simulink model "ADIA"  (R2018b)
settings: Solver=FixedStepDiscrete  StartTime=0.0  StopTime=10.0  FixedStep=0.02  RelTol=1e-3
undefined symbols (not defined in the file or in its folder): ACC_State_Active, ACC_State_BrakeOnly, ACC_State_Suspended, ACC_State_WaitingRise, ADAS_AEBBrakingProg, ADAS_DeclControlReq, ADAS_DriveOff, ADAS_ESCHoldReq_NotHold, ADASDecType_ACC, ADASDecType_AEB, ADIA_ACC_Acceleration_OOR_DecCount_C, ADIA_ACC_Acceleration_OOR_Duration_C, ADIA_ACC_Acceleration_OOR_IncCount_C, ADIA_ACC_Acceleration_OOR_LLim_C, ADIA_ACC_Acceleration_OOR_ULim_C, ADIA_ACC_AccelTrqReq_MixedDia_ULim_C, ADIA_ACC_AccelTrqReq_ULim_C, ADIA_ACC_Deceleration_Mixed_ULim_C, ADIA_ACC_Deceleration_OOR_DecCount_C, ADIA_ACC_Deceleration_OOR_Duration_C, ADIA_ACC_Deceleration_OOR_IncCount_C, ADIA_ACC_Deceleration_OOR_LLim_C, ADIA_ACC_Deceleration_OOR_ULim_C, ADIA_ACC_DriveOff_Distance_C, ADIA_ACC_DriveOff_TimeLim_C, ADIA_ACC_ReqMixed_DecCount_C, ADIA_ACC_ReqMixed_Duration_C, ADIA_ACC_ReqMixed_IncCount_C, ADIA_AccPedalRaw_MaxLim_C, ADIA_AccPedalRaw_MinLim_C, ADIA_ADAS_HoldDecReq_Set_C, ADIA_ADAS_HoldRConfirm_TimeLim_C, ADIA_ADAS_HoldVehSpd_Lim_C, ADIA_AEB_VehSpdDec_LLim_C, ADIA_AEB_VehSpdDec_ULim_C, ADIA_ASWFault_OvrdEn_C, ADIA_ASWFault_OvrdValue_C, ADIA_BatteryOutOfRange_DecCount_C, ADIA_BatteryOutOfRange_Duration_C, ADIA_BatteryOutOfRange_IncCount_C, ADIA_BattVolt_MaxLim_C, ADIA_BattVolt_MinLim_C, ADIA_BCM3_33C_InvBrkLight_DecCount_C, ADIA_BCM3_33C_InvBrkLight_Duration_C, ADIA_BCM3_33C_InvBrkLight_IncCount_C, ADIA_BCM_BattVolt_OvrdEn_C, ADIA_BCM_BattVolt_OvrdVal_C, ADIA_BCM_BrakeLampStaus_OvrdEn_C, ADIA_BCM_BrakeLampStaus_OvrdVal_C, ADIA_BCM_CHMSLStaus_OvrdEn_C, ADIA_BCM_CHMSLStaus_OvrdVal_C, ADIA_BCM_LeftTurnSwSt_OvrdEn_C, ADIA_BCM_LeftTurnSwSt_OvrdVal_C, ADIA_BCM_RightTurnSwSt_OvrdEn_C, ADIA_BCM_RightTurnSwSt_OvrdVal_C, ADIA_BCM_TurnSwFailure_DecCount_C, ADIA_BCM_TurnSwFailure_Duration_C, ADIA_BCM_TurnSwFailure_IncCount_C, ADIA_BSWFault_Ignore_C, ADIA_BSWFault_OvrdEn_C ... (+281)
libraries: simulink x208
(part 8 of 10)

== system ADIA/ADAS_Diagnostics/Diagnostics_Processing/Subsystem3/16Bits_Set1/8Bits_Set1 ==
  Bit1 : Inport  OutDataTypeStr=boolean
  Bit2 : Inport  Port=2  OutDataTypeStr=boolean
  Bit3 : Inport  Port=3  OutDataTypeStr=boolean
  Bit4 : Inport  Port=4  OutDataTypeStr=boolean
  Bit5 : Inport  Port=5  OutDataTypeStr=boolean
  Bit6 : Inport  Port=6  OutDataTypeStr=boolean
  Bit7 : Inport  Port=7  OutDataTypeStr=boolean
  Bit8 : Inport  Port=8  OutDataTypeStr=boolean
  Bit Clear : simulink/Logic and Bit Operations/Bit Clear  iBit=0
      settings: SourceProductName=Simulink  SourceProductBaseCode=SL
  Bit Clear1 : simulink/Logic and Bit Operations/Bit Clear  iBit=1
      settings: SourceProductName=Simulink  SourceProductBaseCode=SL
  Bit Clear2 : simulink/Logic and Bit Operations/Bit Clear  iBit=2
      settings: SourceProductName=Simulink  SourceProductBaseCode=SL
  Bit Clear3 : simulink/Logic and Bit Operations/Bit Clear  iBit=3
      settings: SourceProductName=Simulink  SourceProductBaseCode=SL
  Bit Clear4 : simulink/Logic and Bit Operations/Bit Clear  iBit=5
      settings: SourceProductName=Simulink  SourceProductBaseCode=SL
  Bit Clear5 : simulink/Logic and Bit Operations/Bit Clear  iBit=4
      settings: SourceProductName=Simulink  SourceProductBaseCode=SL
  Bit Clear6 : simulink/Logic and Bit Operations/Bit Clear  iBit=6
      settings: SourceProductName=Simulink  SourceProductBaseCode=SL
  Bit Clear7 : simulink/Logic and Bit Operations/Bit Clear  iBit=7
      settings: SourceProductName=Simulink  SourceProductBaseCode=SL
  Bit Set : simulink/Logic and Bit Operations/Bit Set  iBit=0
      settings: SourceProductName=Simulink  SourceProductBaseCode=SL
  Bit Set1 : simulink/Logic and Bit Operations/Bit Set  iBit=1
      settings: SourceProductName=Simulink  SourceProductBaseCode=SL
  Bit Set2 : simulink/Logic and Bit Operations/Bit Set  iBit=2
      settings: SourceProductName=Simulink  SourceProductBaseCode=SL
  Bit Set3 : simulink/Logic and Bit Operations/Bit Set  iBit=3
      settings: SourceProductName=Simulink  SourceProductBaseCode=SL
  Bit Set4 : simulink/Logic and Bit Operations/Bit Set  iBit=4
      settings: SourceProductName=Simulink  SourceProductBaseCode=SL
  Bit Set5 : simulink/Logic and Bit Operations/Bit Set  iBit=5
      settings: SourceProductName=Simulink  SourceProductBaseCode=SL
  Bit Set6 : simulink/Logic and Bit Operations/Bit Set  iBit=6
      settings: SourceProductName=Simulink  SourceProductBaseCode=SL
  Bit Set7 : simulink/Logic and Bit Operations/Bit Set  iBit=7
      settings: SourceProductName=Simulink  SourceProductBaseCode=SL
  Delay : Delay  DelayLength=1  InitialCondition=0
  Switch{1..8} (8 alike) : Switch  Criteria=u2 > Threshold
  Index_8Bits : Outport  OutDataTypeStr=uint8
  wires:
  Bit Clear7/1 -> Switch8/3
  Bit Clear6/1 -> Switch7/3
  Bit Clear5/1 -> Switch5/3
  Bit Clear4/1 -> Switch6/3
  Bit Clear3/1 -> Switch4/3
  Bit Clear2/1 -> Switch3/3
  Bit Clear1/1 -> Switch2/3
  Bit Clear/1 -> Switch1/3
  Bit Set4/1 -> Switch5/1
  Bit Set2/1 -> Switch3/1
  Switch4/1 -> Bit Set4/1, Bit Clear5/1
  Switch6/1 -> Bit Set6/1, Bit Clear6/1
  Bit Set5/1 -> Switch6/1
  Switch7/1 -> Bit Set7/1, Bit Clear7/1
  Switch2/1 -> Bit Set2/1, Bit Clear2/1
  Bit Set3/1 -> Switch4/1
  Bit Set/1 -> Switch1/1
  Switch3/1 -> Bit Set3/1, Bit Clear3/1
  Bit7/1 -> Switch7/2
  Bit8/1 -> Switch8/2
  Bit Set6/1 -> Switch7/1
  Bit5/1 -> Switch5/2
  Bit6/1 -> Switch6/2
  Bit3/1 -> Switch3/2
  Bit Set1/1 -> Switch2/1
  Delay/1 -> Bit Set/1, Bit Clear/1
  Switch5/1 -> Bit Set5/1, Bit Clear4/1
  Bit2/1 -> Switch2/2
  Switch1/1 -> Bit Set1/1, Bit Clear1/1
  Switch8/1 -> Delay/1, Index_8Bits/1
  Bit4/1 -> Switch4/2
  Bit1/1 -> Switch1/2
  Bit Set7/1 -> Switch8/1

== system ADIA/ADAS_Diagnostics/Diagnostics_Processing/Rationality_Diagnostics/BatteryOutOfRange/Counter&Latch/Latch  ==
  Input : Inport
  Latch Reset : Inport  Port=2
  Constant11 : Constant  Value=0  OutDataTypeStr=Inherit: Inherit via back propagation
  Constant12 : Constant  OutDataTypeStr=Inherit: Inherit via back propagation
  Switch : Switch  Threshold=1  OutDataTypeStr=Inherit: Inherit via back propagation  SaturateOnIntegerOverflow=on  InputSameDT=on
  Switch1 : Switch  Threshold=1  OutDataTypeStr=Inherit: Inherit via back propagation  SaturateOnIntegerOverflow=on  InputSameDT=on
  Unit Delay1 : UnitDelay  SampleTime=-1
  Output : Outport  InitialOutput=0
  wires:
  Constant12/1 -> Switch1/1
  Constant11/1 -> Switch/1
  Input/1 -> Switch1/2
  Unit Delay1/1 -> Switch1/3
  Switch/1 -> Unit Delay1/1, Output/1
  Latch Reset/1 -> Switch/2
  Switch1/1 -> Switch/3

== system ADIA/ADAS_Diagnostics/Diagnostics_Processing/Rationality_Diagnostics/BatteryOutOfRange/Counter&Latch/Timer1 ==
  incrcondition : Inport
  incrvalue : Inport  Port=2
  decrcondition : Inport  Port=3
  decvalue : Inport  Port=4
  maxlimit : Inport  Port=5
  reset : Inport  Port=6
  Constant{,1..3} (4 alike) : Constant  Value=0  OutDataTypeStr=Inherit: Inherit via back propagation
  MinMax1 : MinMax  Inputs=2  OutDataTypeStr=Inherit: Inherit via back propagation  InputSameDT=on
  MinMax2 : MinMax  Function=max  Inputs=2  OutDataTypeStr=Inherit: Inherit via back propagation  InputSameDT=on
  Relational Operator : RelationalOperator  OutDataTypeStr=boolean  RndMeth=Nearest
  Sum : Sum  Inputs=++-  OutDataTypeStr=Inherit: Inherit via back propagation  InputSameDT=on
  Unit Delay : UnitDelay  SampleTime=-1
  dec switch : Switch  Criteria=u2 ~= 0  Threshold=1  OutDataTypeStr=Inherit: Inherit via back propagation  InputSameDT=on
  inc switch : Switch  Criteria=u2 ~= 0  Threshold=1  OutDataTypeStr=Inherit: Inherit via back propagation  InputSameDT=on
  reset switch : Switch  Criteria=u2 ~= 0  Threshold=1  OutDataTypeStr=Inherit: Inherit via back propagation  InputSameDT=on
  counter out : Outport
  counter_status : Outport  Port=2
  wires:
  decvalue/1 -> dec switch/1
  Relational Operator/1 -> counter_status/1
  Constant3/1 -> reset switch/1
  inc switch/1 -> Sum/2
  Sum/1 -> MinMax2/2
  maxlimit/1 -> MinMax1/2, Relational Operator/2
  Constant2/1 -> MinMax2/1
  reset switch/1 -> counter out/1, Relational Operator/1, Unit Delay/1
  Unit Delay/1 -> Sum/1
  reset/1 -> reset switch/2
  Constant/1 -> inc switch/3
  MinMax2/1 -> MinMax1/1
  incrvalue/1 -> inc switch/1
  MinMax1/1 -> reset switch/3
  dec switch/1 -> Sum/3
  Constant1/1 -> dec switch/3
  decrcondition/1 -> dec switch/2
  incrcondition/1 -> inc switch/2

== system ADIA/ADAS_Diagnostics/Diagnostics_Processing/Rationality_Diagnostics/CameraSystemError/Counter&Latch/Latch  ==
  Input : Inport
  Latch Reset : Inport  Port=2
  Constant11 : Constant  Value=0  OutDataTypeStr=Inherit: Inherit via back propagation
  Constant12 : Constant  OutDataTypeStr=Inherit: Inherit via back propagation
  Switch : Switch  Threshold=1  OutDataTypeStr=Inherit: Inherit via back propagation  SaturateOnIntegerOverflow=on  InputSameDT=on
  Switch1 : Switch  Threshold=1  OutDataTypeStr=Inherit: Inherit via back propagation  SaturateOnIntegerOverflow=on  InputSameDT=on
  Unit Delay1 : UnitDelay  SampleTime=-1
  Output : Outport  InitialOutput=0
  wires:
  Constant12/1 -> Switch1/1
  Constant11/1 -> Switch/1
  Input/1 -> Switch1/2
  Unit Delay1/1 -> Switch1/3
  Switch/1 -> Unit Delay1/1, Output/1
  Latch Reset/1 -> Switch/2
  Switch1/1 -> Switch/3

== system ADIA/ADAS_Diagnostics/Diagnostics_Processing/Rationality_Diagnostics/CameraSystemError/Counter&Latch/Timer1 ==
  incrcondition : Inport
  incrvalue : Inport  Port=2
  decrcondition : Inport  Port=3
  decvalue : Inport  Port=4
  maxlimit : Inport  Port=5
  reset : Inport  Port=6
  Constant{,1..3} (4 alike) : Constant  Value=0  OutDataTypeStr=Inherit: Inherit via back propagation
  MinMax1 : MinMax  Inputs=2  OutDataTypeStr=Inherit: Inherit via back propagation  InputSameDT=on
  MinMax2 : MinMax  Function=max  Inputs=2  OutDataTypeStr=Inherit: Inherit via back propagation  InputSameDT=on
  Relational Operator : RelationalOperator  OutDataTypeStr=boolean  RndMeth=Nearest
  Sum : Sum  Inputs=++-  OutDataTypeStr=Inherit: Inherit via back propagation  InputSameDT=on
  Unit Delay : UnitDelay  SampleTime=-1
  dec switch : Switch  Criteria=u2 ~= 0  Threshold=1  OutDataTypeStr=Inherit: Inherit via back propagation  InputSameDT=on
  inc switch : Switch  Criteria=u2 ~= 0  Threshold=1  OutDataTypeStr=Inherit: Inherit via back propagation  InputSameDT=on
  reset switch : Switch  Criteria=u2 ~= 0  Threshold=1  OutDataTypeStr=Inherit: Inherit via back propagation  InputSameDT=on
  counter out : Outport
  counter_status : Outport  Port=2
  wires:
  decvalue/1 -> dec switch/1
  Relational Operator/1 -> counter_status/1
  Constant3/1 -> reset switch/1
  inc switch/1 -> Sum/2
  Sum/1 -> MinMax2/2
  maxlimit/1 -> MinMax1/2, Relational Operator/2
  Constant2/1 -> MinMax2/1
  reset switch/1 -> counter out/1, Relational Operator/1, Unit Delay/1
  Unit Delay/1 -> Sum/1
  reset/1 -> reset switch/2
  Constant/1 -> inc switch/3
  MinMax2/1 -> MinMax1/1
  incrvalue/1 -> inc switch/1
  MinMax1/1 -> reset switch/3
  dec switch/1 -> Sum/3
  Constant1/1 -> dec switch/3
  decrcondition/1 -> dec switch/2
  incrcondition/1 -> inc switch/2

== system ADIA/ADAS_Diagnostics/Diagnostics_Processing/Rationality_Diagnostics/DTC_BCM3_33C_InvBrkLight/Counter&Latch/Latch  ==
  Input : Inport
  Latch Reset : Inport  Port=2
  Constant11 : Constant  Value=0  OutDataTypeStr=Inherit: Inherit via back propagation
  Constant12 : Constant  OutDataTypeStr=Inherit: Inherit via back propagation
  Switch : Switch  Threshold=1  OutDataTypeStr=Inherit: Inherit via back propagation  SaturateOnIntegerOverflow=on  InputSameDT=on
  Switch1 : Switch  Threshold=1  OutDataTypeStr=Inherit: Inherit via back propagation  SaturateOnIntegerOverflow=on  InputSameDT=on
  Unit Delay1 : UnitDelay  SampleTime=-1
  Output : Outport  InitialOutput=0
  wires:
  Constant12/1 -> Switch1/1
  Constant11/1 -> Switch/1
  Input/1 -> Switch1/2
  Unit Delay1/1 -> Switch1/3
  Switch/1 -> Unit Delay1/1, Output/1
  Latch Reset/1 -> Switch/2
  Switch1/1 -> Switch/3

== system ADIA/ADAS_Diagnostics/Diagnostics_Processing/Rationality_Diagnostics/DTC_BCM3_33C_InvBrkLight/Counter&Latch/Timer1 ==
  incrcondition : Inport
  incrvalue : Inport  Port=2
  decrcondition : Inport  Port=3
  decvalue : Inport  Port=4
  maxlimit : Inport  Port=5
  reset : Inport  Port=6
  Constant{,1..3} (4 alike) : Constant  Value=0  OutDataTypeStr=Inherit: Inherit via back propagation
  MinMax1 : MinMax  Inputs=2  OutDataTypeStr=Inherit: Inherit via back propagation  InputSameDT=on
  MinMax2 : MinMax  Function=max  Inputs=2  OutDataTypeStr=Inherit: Inherit via back propagation  InputSameDT=on
  Relational Operator : RelationalOperator  OutDataTypeStr=boolean  RndMeth=Nearest
  Sum : Sum  Inputs=++-  OutDataTypeStr=Inherit: Inherit via back propagation  InputSameDT=on
  Unit Delay : UnitDelay  SampleTime=-1
  dec switch : Switch  Criteria=u2 ~= 0  Threshold=1  OutDataTypeStr=Inherit: Inherit via back propagation  InputSameDT=on
  inc switch : Switch  Criteria=u2 ~= 0  Threshold=1  OutDataTypeStr=Inherit: Inherit via back propagation  InputSameDT=on
  reset switch : Switch  Criteria=u2 ~= 0  Threshold=1  OutDataTypeStr=Inherit: Inherit via back propagation  InputSameDT=on
  counter out : Outport
  counter_status : Outport  Port=2
  wires:
  decvalue/1 -> dec switch/1
  Relational Operator/1 -> counter_status/1
  Constant3/1 -> reset switch/1
  inc switch/1 -> Sum/2
  Sum/1 -> MinMax2/2
  maxlimit/1 -> MinMax1/2, Relational Operator/2
  Constant2/1 -> MinMax2/1
  reset switch/1 -> counter out/1, Relational Operator/1, Unit Delay/1
  Unit Delay/1 -> Sum/1
  reset/1 -> reset switch/2
  Constant/1 -> inc switch/3
  MinMax2/1 -> MinMax1/1
  incrvalue/1 -> inc switch/1
  MinMax1/1 -> reset switch/3
  dec switch/1 -> Sum/3
  Constant1/1 -> dec switch/3
  decrcondition/1 -> dec switch/2
  incrcondition/1 -> inc switch/2

== system ADIA/ADAS_Diagnostics/Diagnostics_Processing/Rationality_Diagnostics/DTC_EMS_14A_OorACCStatus/Counter&Latch/Latch  ==
  Input : Inport
  Latch Reset : Inport  Port=2
  Constant11 : Constant  Value=0  OutDataTypeStr=Inherit: Inherit via back propagation
  Constant12 : Constant  OutDataTypeStr=Inherit: Inherit via back propagation
  Switch : Switch  Threshold=1  OutDataTypeStr=Inherit: Inherit via back propagation  SaturateOnIntegerOverflow=on  InputSameDT=on
  Switch1 : Switch  Threshold=1  OutDataTypeStr=Inherit: Inherit via back propagation  SaturateOnIntegerOverflow=on  InputSameDT=on
  Unit Delay1 : UnitDelay  SampleTime=-1
  Output : Outport  InitialOutput=0
  wires:
  Constant12/1 -> Switch1/1
  Constant11/1 -> Switch/1
  Input/1 -> Switch1/2
  Unit Delay1/1 -> Switch1/3
  Switch/1 -> Unit Delay1/1, Output/1
  Latch Reset/1 -> Switch/2
  Switch1/1 -> Switch/3

== system ADIA/ADAS_Diagnostics/Diagnostics_Processing/Rationality_Diagnostics/DTC_EMS_14A_OorACCStatus/Counter&Latch/Timer1 ==
  incrcondition : Inport
  incrvalue : Inport  Port=2
  decrcondition : Inport  Port=3
  decvalue : Inport  Port=4
  maxlimit : Inport  Port=5
  reset : Inport  Port=6
  Constant{,1..3} (4 alike) : Constant  Value=0  OutDataTypeStr=Inherit: Inherit via back propagation
  MinMax1 : MinMax  Inputs=2  OutDataTypeStr=Inherit: Inherit via back propagation  InputSameDT=on
  MinMax2 : MinMax  Function=max  Inputs=2  OutDataTypeStr=Inherit: Inherit via back propagation  InputSameDT=on
  Relational Operator : RelationalOperator  OutDataTypeStr=boolean  RndMeth=Nearest
  Sum : Sum  Inputs=++-  OutDataTypeStr=Inherit: Inherit via back propagation  InputSameDT=on
  Unit Delay : UnitDelay  SampleTime=-1
  dec switch : Switch  Criteria=u2 ~= 0  Threshold=1  OutDataTypeStr=Inherit: Inherit via back propagation  InputSameDT=on
  inc switch : Switch  Criteria=u2 ~= 0  Threshold=1  OutDataTypeStr=Inherit: Inherit via back propagation  InputSameDT=on
  reset switch : Switch  Criteria=u2 ~= 0  Threshold=1  OutDataTypeStr=Inherit: Inherit via back propagation  InputSameDT=on
  counter out : Outport
  counter_status : Outport  Port=2
  wires:
  decvalue/1 -> dec switch/1
  Relational Operator/1 -> counter_status/1
  Constant3/1 -> reset switch/1
  inc switch/1 -> Sum/2
  Sum/1 -> MinMax2/2
  maxlimit/1 -> MinMax1/2, Relational Operator/2
  Constant2/1 -> MinMax2/1
  reset switch/1 -> counter out/1, Relational Operator/1, Unit Delay/1
  Unit Delay/1 -> Sum/1
  reset/1 -> reset switch/2
  Constant/1 -> inc switch/3
  MinMax2/1 -> MinMax1/1
  incrvalue/1 -> inc switch/1
  MinMax1/1 -> reset switch/3
  dec switch/1 -> Sum/3
  Constant1/1 -> dec switch/3
  decrcondition/1 -> dec switch/2
  incrcondition/1 -> inc switch/2

== system ADIA/ADAS_Diagnostics/Diagnostics_Processing/Rationality_Diagnostics/DTC_WheelSpdFaultSignal/Counter&Latch/Latch  ==
  Input : Inport
  Latch Reset : Inport  Port=2
  Constant11 : Constant  Value=0  OutDataTypeStr=Inherit: Inherit via back propagation
  Constant12 : Constant  OutDataTypeStr=Inherit: Inherit via back propagation
  Switch : Switch  Threshold=1  OutDataTypeStr=Inherit: Inherit via back propagation  SaturateOnIntegerOverflow=on  InputSameDT=on
  Switch1 : Switch  Threshold=1  OutDataTypeStr=Inherit: Inherit via back propagation  SaturateOnIntegerOverflow=on  InputSameDT=on
  Unit Delay1 : UnitDelay  SampleTime=-1
  Output : Outport  InitialOutput=0
  wires:
  Constant12/1 -> Switch1/1
  Constant11/1 -> Switch/1
  Input/1 -> Switch1/2
  Unit Delay1/1 -> Switch1/3
  Switch/1 -> Unit Delay1/1, Output/1
  Latch Reset/1 -> Switch/2
  Switch1/1 -> Switch/3

== system ADIA/ADAS_Diagnostics/Diagnostics_Processing/Rationality_Diagnostics/DTC_WheelSpdFaultSignal/Counter&Latch/Timer1 ==
  incrcondition : Inport
  incrvalue : Inport  Port=2
  decrcondition : Inport  Port=3
  decvalue : Inport  Port=4
  maxlimit : Inport  Port=5
  reset : Inport  Port=6
  Constant{,1..3} (4 alike) : Constant  Value=0  OutDataTypeStr=Inherit: Inherit via back propagation
  MinMax1 : MinMax  Inputs=2  OutDataTypeStr=Inherit: Inherit via back propagation  InputSameDT=on
  MinMax2 : MinMax  Function=max  Inputs=2  OutDataTypeStr=Inherit: Inherit via back propagation  InputSameDT=on
  Relational Operator : RelationalOperator  OutDataTypeStr=boolean  RndMeth=Nearest
  Sum : Sum  Inputs=++-  OutDataTypeStr=Inherit: Inherit via back propagation  InputSameDT=on
  Unit Delay : UnitDelay  SampleTime=-1
  dec switch : Switch  Criteria=u2 ~= 0  Threshold=1  OutDataTypeStr=Inherit: Inherit via back propagation  InputSameDT=on
  inc switch : Switch  Criteria=u2 ~= 0  Threshold=1  OutDataTypeStr=Inherit: Inherit via back propagation  InputSameDT=on
  reset switch : Switch  Criteria=u2 ~= 0  Threshold=1  OutDataTypeStr=Inherit: Inherit via back propagation  InputSameDT=on
  counter out : Outport
  counter_status : Outport  Port=2
  wires:
  decvalue/1 -> dec switch/1
  Relational Operator/1 -> counter_status/1
  Constant3/1 -> reset switch/1
  inc switch/1 -> Sum/2
  Sum/1 -> MinMax2/2
  maxlimit/1 -> MinMax1/2, Relational Operator/2
  Constant2/1 -> MinMax2/1
  reset switch/1 -> counter out/1, Relational Operator/1, Unit Delay/1
  Unit Delay/1 -> Sum/1
  reset/1 -> reset switch/2
  Constant/1 -> inc switch/3
  MinMax2/1 -> MinMax1/1
  incrvalue/1 -> inc switch/1
  MinMax1/1 -> reset switch/3
  dec switch/1 -> Sum/3
  Constant1/1 -> dec switch/3
  decrcondition/1 -> dec switch/2
  incrcondition/1 -> inc switch/2

== system ADIA/ADAS_Diagnostics/Diagnostics_Processing/Rationality_Diagnostics/EMS10_88_InvAccPedPosRaw/Counter&Latch/Latch  ==
  Input : Inport
  Latch Reset : Inport  Port=2
  Constant11 : Constant  Value=0  OutDataTypeStr=Inherit: Inherit via back propagation
  Constant12 : Constant  OutDataTypeStr=Inherit: Inherit via back propagation
  Switch : Switch  Threshold=1  OutDataTypeStr=Inherit: Inherit via back propagation  SaturateOnIntegerOverflow=on  InputSameDT=on
  Switch1 : Switch  Threshold=1  OutDataTypeStr=Inherit: Inherit via back propagation  SaturateOnIntegerOverflow=on  InputSameDT=on
  Unit Delay1 : UnitDelay  SampleTime=-1
  Output : Outport  InitialOutput=0
  wires:
  Constant12/1 -> Switch1/1
  Constant11/1 -> Switch/1
  Input/1 -> Switch1/2
  Unit Delay1/1 -> Switch1/3
  Switch/1 -> Unit Delay1/1, Output/1
  Latch Reset/1 -> Switch/2
  Switch1/1 -> Switch/3

== system ADIA/ADAS_Diagnostics/Diagnostics_Processing/Rationality_Diagnostics/EMS10_88_InvAccPedPosRaw/Counter&Latch/Timer1 ==
  incrcondition : Inport
  incrvalue : Inport  Port=2
  decrcondition : Inport  Port=3
  decvalue : Inport  Port=4
  maxlimit : Inport  Port=5
  reset : Inport  Port=6
  Constant{,1..3} (4 alike) : Constant  Value=0  OutDataTypeStr=Inherit: Inherit via back propagation
  MinMax1 : MinMax  Inputs=2  OutDataTypeStr=Inherit: Inherit via back propagation  InputSameDT=on
  MinMax2 : MinMax  Function=max  Inputs=2  OutDataTypeStr=Inherit: Inherit via back propagation  InputSameDT=on
  Relational Operator : RelationalOperator  OutDataTypeStr=boolean  RndMeth=Nearest
  Sum : Sum  Inputs=++-  OutDataTypeStr=Inherit: Inherit via back propagation  InputSameDT=on
  Unit Delay : UnitDelay  SampleTime=-1
  dec switch : Switch  Criteria=u2 ~= 0  Threshold=1  OutDataTypeStr=Inherit: Inherit via back propagation  InputSameDT=on
  inc switch : Switch  Criteria=u2 ~= 0  Threshold=1  OutDataTypeStr=Inherit: Inherit via back propagation  InputSameDT=on
  reset switch : Switch  Criteria=u2 ~= 0  Threshold=1  OutDataTypeStr=Inherit: Inherit via back propagation  InputSameDT=on
  counter out : Outport
  counter_status : Outport  Port=2
  wires:
  decvalue/1 -> dec switch/1
  Relational Operator/1 -> counter_status/1
  Constant3/1 -> reset switch/1
  inc switch/1 -> Sum/2
  Sum/1 -> MinMax2/2
  maxlimit/1 -> MinMax1/2, Relational Operator/2
  Constant2/1 -> MinMax2/1
  reset switch/1 -> counter out/1, Relational Operator/1, Unit Delay/1
  Unit Delay/1 -> Sum/1
  reset/1 -> reset switch/2
  Constant/1 -> inc switch/3
  MinMax2/1 -> MinMax1/1
  incrvalue/1 -> inc switch/1
  MinMax1/1 -> reset switch/3
  dec switch/1 -> Sum/3
  Constant1/1 -> dec switch/3
  decrcondition/1 -> dec switch/2
  incrcondition/1 -> inc switch/2

== system ADIA/ADAS_Diagnostics/Diagnostics_Processing/Rationality_Diagnostics/EMS5_E0_InvOorBrkPedal/Counter&Latch/Latch  ==
  Input : Inport
  Latch Reset : Inport  Port=2
  Constant11 : Constant  Value=0  OutDataTypeStr=Inherit: Inherit via back propagation
  Constant12 : Constant  OutDataTypeStr=Inherit: Inherit via back propagation
  Switch : Switch  Threshold=1  OutDataTypeStr=Inherit: Inherit via back propagation  SaturateOnIntegerOverflow=on  InputSameDT=on
  Switch1 : Switch  Threshold=1  OutDataTypeStr=Inherit: Inherit via back propagation  SaturateOnIntegerOverflow=on  InputSameDT=on
  Unit Delay1 : UnitDelay  SampleTime=-1
  Output : Outport  InitialOutput=0
  wires:
  Constant12/1 -> Switch1/1
  Constant11/1 -> Switch/1
  Input/1 -> Switch1/2
  Unit Delay1/1 -> Switch1/3
  Switch/1 -> Unit Delay1/1, Output/1
  Latch Reset/1 -> Switch/2
  Switch1/1 -> Switch/3

== system ADIA/ADAS_Diagnostics/Diagnostics_Processing/Rationality_Diagnostics/EMS5_E0_InvOorBrkPedal/Counter&Latch/Timer1 ==
  incrcondition : Inport
  incrvalue : Inport  Port=2
  decrcondition : Inport  Port=3
  decvalue : Inport  Port=4
  maxlimit : Inport  Port=5
  reset : Inport  Port=6
  Constant{,1..3} (4 alike) : Constant  Value=0  OutDataTypeStr=Inherit: Inherit via back propagation
  MinMax1 : MinMax  Inputs=2  OutDataTypeStr=Inherit: Inherit via back propagation  InputSameDT=on
  MinMax2 : MinMax  Function=max  Inputs=2  OutDataTypeStr=Inherit: Inherit via back propagation  InputSameDT=on
  Relational Operator : RelationalOperator  OutDataTypeStr=boolean  RndMeth=Nearest
  Sum : Sum  Inputs=++-  OutDataTypeStr=Inherit: Inherit via back propagation  InputSameDT=on
  Unit Delay : UnitDelay  SampleTime=-1
  dec switch : Switch  Criteria=u2 ~= 0  Threshold=1  OutDataTypeStr=Inherit: Inherit via back propagation  InputSameDT=on
  inc switch : Switch  Criteria=u2 ~= 0  Threshold=1  OutDataTypeStr=Inherit: Inherit via back propagation  InputSameDT=on
  reset switch : Switch  Criteria=u2 ~= 0  Threshold=1  OutDataTypeStr=Inherit: Inherit via back propagation  InputSameDT=on
  counter out : Outport
  counter_status : Outport  Port=2
  wires:
  decvalue/1 -> dec switch/1
  Relational Operator/1 -> counter_status/1
  Constant3/1 -> reset switch/1
  inc switch/1 -> Sum/2
  Sum/1 -> MinMax2/2
  maxlimit/1 -> MinMax1/2, Relational Operator/2
  Constant2/1 -> MinMax2/1
  reset switch/1 -> counter out/1, Relational Operator/1, Unit Delay/1
  Unit Delay/1 -> Sum/1
  reset/1 -> reset switch/2
  Constant/1 -> inc switch/3
  MinMax2/1 -> MinMax1/1
  incrvalue/1 -> inc switch/1
  MinMax1/1 -> reset switch/3
  dec switch/1 -> Sum/3
  Constant1/1 -> dec switch/3
  decrcondition/1 -> dec switch/2
  incrcondition/1 -> inc switch/2

== system ADIA/ADAS_Diagnostics/Diagnostics_Processing/Rationality_Diagnostics/EMS5_E0_OorEngineStas/Counter&Latch/Latch  ==
  Input : Inport
  Latch Reset : Inport  Port=2
  Constant11 : Constant  Value=0  OutDataTypeStr=Inherit: Inherit via back propagation
  Constant12 : Constant  OutDataTypeStr=Inherit: Inherit via back propagation
  Switch : Switch  Threshold=1  OutDataTypeStr=Inherit: Inherit via back propagation  SaturateOnIntegerOverflow=on  InputSameDT=on
  Switch1 : Switch  Threshold=1  OutDataTypeStr=Inherit: Inherit via back propagation  SaturateOnIntegerOverflow=on  InputSameDT=on
  Unit Delay1 : UnitDelay  SampleTime=-1
  Output : Outport  InitialOutput=0
  wires:
  Constant12/1 -> Switch1/1
  Constant11/1 -> Switch/1
  Input/1 -> Switch1/2
  Unit Delay1/1 -> Switch1/3
  Switch/1 -> Unit Delay1/1, Output/1
  Latch Reset/1 -> Switch/2
  Switch1/1 -> Switch/3

== system ADIA/ADAS_Diagnostics/Diagnostics_Processing/Rationality_Diagnostics/EMS5_E0_OorEngineStas/Counter&Latch/Timer1 ==
  incrcondition : Inport
  incrvalue : Inport  Port=2
  decrcondition : Inport  Port=3
  decvalue : Inport  Port=4
  maxlimit : Inport  Port=5
  reset : Inport  Port=6
  Constant{,1..3} (4 alike) : Constant  Value=0  OutDataTypeStr=Inherit: Inherit via back propagation
  MinMax1 : MinMax  Inputs=2  OutDataTypeStr=Inherit: Inherit via back propagation  InputSameDT=on
  MinMax2 : MinMax  Function=max  Inputs=2  OutDataTypeStr=Inherit: Inherit via back propagation  InputSameDT=on
  Relational Operator : RelationalOperator  OutDataTypeStr=boolean  RndMeth=Nearest
  Sum : Sum  Inputs=++-  OutDataTypeStr=Inherit: Inherit via back propagation  InputSameDT=on
  Unit Delay : UnitDelay  SampleTime=-1
  dec switch : Switch  Criteria=u2 ~= 0  Threshold=1  OutDataTypeStr=Inherit: Inherit via back propagation  InputSameDT=on
  inc switch : Switch  Criteria=u2 ~= 0  Threshold=1  OutDataTypeStr=Inherit: Inherit via back propagation  InputSameDT=on
  reset switch : Switch  Criteria=u2 ~= 0  Threshold=1  OutDataTypeStr=Inherit: Inherit via back propagation  InputSameDT=on
  counter out : Outport
  counter_status : Outport  Port=2
  wires:
  decvalue/1 -> dec switch/1
  Relational Operator/1 -> counter_status/1
  Constant3/1 -> reset switch/1
  inc switch/1 -> Sum/2
  Sum/1 -> MinMax2/2
  maxlimit/1 -> MinMax1/2, Relational Operator/2
  Constant2/1 -> MinMax2/1
  reset switch/1 -> counter out/1, Relational Operator/1, Unit Delay/1
  Unit Delay/1 -> Sum/1
  reset/1 -> reset switch/2
  Constant/1 -> inc switch/3
  MinMax2/1 -> MinMax1/1
  incrvalue/1 -> inc switch/1
  MinMax1/1 -> reset switch/3
  dec switch/1 -> Sum/3
  Constant1/1 -> dec switch/3
  decrcondition/1 -> dec switch/2
  incrcondition/1 -> inc switch/2

== system ADIA/ADAS_Diagnostics/Diagnostics_Processing/Rationality_Diagnostics/EMS_14B_InvOorRealWhlTrq/Counter&Latch/Latch  ==
  Input : Inport
  Latch Reset : Inport  Port=2
  Constant11 : Constant  Value=0  OutDataTypeStr=Inherit: Inherit via back propagation
  Constant12 : Constant  OutDataTypeStr=Inherit: Inherit via back propagation
  Switch : Switch  Threshold=1  OutDataTypeStr=Inherit: Inherit via back propagation  SaturateOnIntegerOverflow=on  InputSameDT=on
  Switch1 : Switch  Threshold=1  OutDataTypeStr=Inherit: Inherit via back propagation  SaturateOnIntegerOverflow=on  InputSameDT=on
  Unit Delay1 : UnitDelay  SampleTime=-1
  Output : Outport  InitialOutput=0
  wires:
  Constant12/1 -> Switch1/1
  Constant11/1 -> Switch/1
  Input/1 -> Switch1/2
  Unit Delay1/1 -> Switch1/3
  Switch/1 -> Unit Delay1/1, Output/1
  Latch Reset/1 -> Switch/2
  Switch1/1 -> Switch/3

== system ADIA/ADAS_Diagnostics/Diagnostics_Processing/Rationality_Diagnostics/EMS_14B_InvOorRealWhlTrq/Counter&Latch/Timer1 ==
  incrcondition : Inport
  incrvalue : Inport  Port=2
  decrcondition : Inport  Port=3
  decvalue : Inport  Port=4
  maxlimit : Inport  Port=5
  reset : Inport  Port=6
  Constant{,1..3} (4 alike) : Constant  Value=0  OutDataTypeStr=Inherit: Inherit via back propagation
  MinMax1 : MinMax  Inputs=2  OutDataTypeStr=Inherit: Inherit via back propagation  InputSameDT=on
  MinMax2 : MinMax  Function=max  Inputs=2  OutDataTypeStr=Inherit: Inherit via back propagation  InputSameDT=on
  Relational Operator : RelationalOperator  OutDataTypeStr=boolean  RndMeth=Nearest
  Sum : Sum  Inputs=++-  OutDataTypeStr=Inherit: Inherit via back propagation  InputSameDT=on
  Unit Delay : UnitDelay  SampleTime=-1
  dec switch : Switch  Criteria=u2 ~= 0  Threshold=1  OutDataTypeStr=Inherit: Inherit via back propagation  InputSameDT=on
  inc switch : Switch  Criteria=u2 ~= 0  Threshold=1  OutDataTypeStr=Inherit: Inherit via back propagation  InputSameDT=on
  reset switch : Switch  Criteria=u2 ~= 0  Threshold=1  OutDataTypeStr=Inherit: Inherit via back propagation  InputSameDT=on
  counter out : Outport
  counter_status : Outport  Port=2
  wires:
  decvalue/1 -> dec switch/1
  Relational Operator/1 -> counter_status/1
  Constant3/1 -> reset switch/1
  inc switch/1 -> Sum/2
  Sum/1 -> MinMax2/2
  maxlimit/1 -> MinMax1/2, Relational Operator/2
  Constant2/1 -> MinMax2/1
  reset switch/1 -> counter out/1, Relational Operator/1, Unit Delay/1
  Unit Delay/1 -> Sum/1
  reset/1 -> reset switch/2
  Constant/1 -> inc switch/3
  MinMax2/1 -> MinMax1/1
  incrvalue/1 -> inc switch/1
  MinMax1/1 -> reset switch/3
  dec switch/1 -> Sum/3
  Constant1/1 -> dec switch/3
  decrcondition/1 -> dec switch/2
  incrcondition/1 -> inc switch/2

== system ADIA/ADAS_Diagnostics/Diagnostics_Processing/Rationality_Diagnostics/EMS_17E_InvOorMaxNoCtrlTrq/Counter&Latch/Latch  ==
  Input : Inport
  Latch Reset : Inport  Port=2
  Constant11 : Constant  Value=0  OutDataTypeStr=Inherit: Inherit via back propagation
  Constant12 : Constant  OutDataTypeStr=Inherit: Inherit via back propagation
  Switch : Switch  Threshold=1  OutDataTypeStr=Inherit: Inherit via back propagation  SaturateOnIntegerOverflow=on  InputSameDT=on
  Switch1 : Switch  Threshold=1  OutDataTypeStr=Inherit: Inherit via back propagation  SaturateOnIntegerOverflow=on  InputSameDT=on
  Unit Delay1 : UnitDelay  SampleTime=-1
  Output : Outport  InitialOutput=0
  wires:
  Constant12/1 -> Switch1/1
  Constant11/1 -> Switch/1
  Input/1 -> Switch1/2
  Unit Delay1/1 -> Switch1/3
  Switch/1 -> Unit Delay1/1, Output/1
  Latch Reset/1 -> Switch/2
  Switch1/1 -> Switch/3

== system ADIA/ADAS_Diagnostics/Diagnostics_Processing/Rationality_Diagnostics/EMS_17E_InvOorMaxNoCtrlTrq/Counter&Latch/Timer1 ==
  incrcondition : Inport
  incrvalue : Inport  Port=2
  decrcondition : Inport  Port=3
  decvalue : Inport  Port=4
  maxlimit : Inport  Port=5
  reset : Inport  Port=6
  Constant{,1..3} (4 alike) : Constant  Value=0  OutDataTypeStr=Inherit: Inherit via back propagation
  MinMax1 : MinMax  Inputs=2  OutDataTypeStr=Inherit: Inherit via back propagation  InputSameDT=on
  MinMax2 : MinMax  Function=max  Inputs=2  OutDataTypeStr=Inherit: Inherit via back propagation  InputSameDT=on
  Relational Operator : RelationalOperator  OutDataTypeStr=boolean  RndMeth=Nearest
  Sum : Sum  Inputs=++-  OutDataTypeStr=Inherit: Inherit via back propagation  InputSameDT=on
  Unit Delay : UnitDelay  SampleTime=-1
  dec switch : Switch  Criteria=u2 ~= 0  Threshold=1  OutDataTypeStr=Inherit: Inherit via back propagation  InputSameDT=on
  inc switch : Switch  Criteria=u2 ~= 0  Threshold=1  OutDataTypeStr=Inherit: Inherit via back propagation  InputSameDT=on
  reset switch : Switch  Criteria=u2 ~= 0  Threshold=1  OutDataTypeStr=Inherit: Inherit via back propagation  InputSameDT=on
  counter out : Outport
  counter_status : Outport  Port=2
  wires:
  decvalue/1 -> dec switch/1
  Relational Operator/1 -> counter_status/1
  Constant3/1 -> reset switch/1
  inc switch/1 -> Sum/2
  Sum/1 -> MinMax2/2
  maxlimit/1 -> MinMax1/2, Relational Operator/2
  Constant2/1 -> MinMax2/1
  reset switch/1 -> counter out/1, Relational Operator/1, Unit Delay/1
  Unit Delay/1 -> Sum/1
  reset/1 -> reset switch/2
  Constant/1 -> inc switch/3
  MinMax2/1 -> MinMax1/1
  incrvalue/1 -> inc switch/1
  MinMax1/1 -> reset switch/3
  dec switch/1 -> Sum/3
  Constant1/1 -> dec switch/3
  decrcondition/1 -> dec switch/2
  incrcondition/1 -> inc switch/2

== system ADIA/ADAS_Diagnostics/Diagnostics_Processing/Rationality_Diagnostics/EMS_17E_InvOorMaxTrqWhl/Counter&Latch/Latch  ==
  Input : Inport
  Latch Reset : Inport  Port=2
  Constant11 : Constant  Value=0  OutDataTypeStr=Inherit: Inherit via back propagation
  Constant12 : Constant  OutDataTypeStr=Inherit: Inherit via back propagation
  Switch : Switch  Threshold=1  OutDataTypeStr=Inherit: Inherit via back propagation  SaturateOnIntegerOverflow=on  InputSameDT=on
  Switch1 : Switch  Threshold=1  OutDataTypeStr=Inherit: Inherit via back propagation  SaturateOnIntegerOverflow=on  InputSameDT=on
  Unit Delay1 : UnitDelay  SampleTime=-1
  Output : Outport  InitialOutput=0
  wires:
  Constant12/1 -> Switch1/1
  Constant11/1 -> Switch/1
  Input/1 -> Switch1/2
  Unit Delay1/1 -> Switch1/3
  Switch/1 -> Unit Delay1/1, Output/1
  Latch Reset/1 -> Switch/2
  Switch1/1 -> Switch/3

== system ADIA/ADAS_Diagnostics/Diagnostics_Processing/Rationality_Diagnostics/EMS_17E_InvOorMaxTrqWhl/Counter&Latch/Timer1 ==
  incrcondition : Inport
  incrvalue : Inport  Port=2
  decrcondition : Inport  Port=3
  decvalue : Inport  Port=4
  maxlimit : Inport  Port=5
  reset : Inport  Port=6
  Constant{,1..3} (4 alike) : Constant  Value=0  OutDataTypeStr=Inherit: Inherit via back propagation
  MinMax1 : MinMax  Inputs=2  OutDataTypeStr=Inherit: Inherit via back propagation  InputSameDT=on
  MinMax2 : MinMax  Function=max  Inputs=2  OutDataTypeStr=Inherit: Inherit via back propagation  InputSameDT=on
  Relational Operator : RelationalOperator  OutDataTypeStr=boolean  RndMeth=Nearest
  Sum : Sum  Inputs=++-  OutDataTypeStr=Inherit: Inherit via back propagation  InputSameDT=on
  Unit Delay : UnitDelay  SampleTime=-1
  dec switch : Switch  Criteria=u2 ~= 0  Threshold=1  OutDataTypeStr=Inherit: Inherit via back propagation  InputSameDT=on
  inc switch : Switch  Criteria=u2 ~= 0  Threshold=1  OutDataTypeStr=Inherit: Inherit via back propagation  InputSameDT=on
  reset switch : Switch  Criteria=u2 ~= 0  Threshold=1  OutDataTypeStr=Inherit: Inherit via back propagation  InputSameDT=on
  counter out : Outport
  counter_status : Outport  Port=2
  wires:
  decvalue/1 -> dec switch/1
  Relational Operator/1 -> counter_status/1
  Constant3/1 -> reset switch/1
  inc switch/1 -> Sum/2
  Sum/1 -> MinMax2/2
  maxlimit/1 -> MinMax1/2, Relational Operator/2
  Constant2/1 -> MinMax2/1
  reset switch/1 -> counter out/1, Relational Operator/1, Unit Delay/1
  Unit Delay/1 -> Sum/1
  reset/1 -> reset switch/2
  Constant/1 -> inc switch/3
  MinMax2/1 -> MinMax1/1
  incrvalue/1 -> inc switch/1
  MinMax1/1 -> reset switch/3
  dec switch/1 -> Sum/3
  Constant1/1 -> dec switch/3
  decrcondition/1 -> dec switch/2
  incrcondition/1 -> inc switch/2

== system ADIA/ADAS_Diagnostics/Diagnostics_Processing/Rationality_Diagnostics/EMS_17E_InvOorMinNoCtrlTrq/Counter&Latch/Latch  ==
  Input : Inport
  Latch Reset : Inport  Port=2
  Constant11 : Constant  Value=0  OutDataTypeStr=Inherit: Inherit via back propagation
  Constant12 : Constant  OutDataTypeStr=Inherit: Inherit via back propagation
  Switch : Switch  Threshold=1  OutDataTypeStr=Inherit: Inherit via back propagation  SaturateOnIntegerOverflow=on  InputSameDT=on
  Switch1 : Switch  Threshold=1  OutDataTypeStr=Inherit: Inherit via back propagation  SaturateOnIntegerOverflow=on  InputSameDT=on
  Unit Delay1 : UnitDelay  SampleTime=-1
  Output : Outport  InitialOutput=0
  wires:
  Constant12/1 -> Switch1/1
  Constant11/1 -> Switch/1
  Input/1 -> Switch1/2
  Unit Delay1/1 -> Switch1/3
  Switch/1 -> Unit Delay1/1, Output/1
  Latch Reset/1 -> Switch/2
  Switch1/1 -> Switch/3

== system ADIA/ADAS_Diagnostics/Diagnostics_Processing/Rationality_Diagnostics/EMS_17E_InvOorMinNoCtrlTrq/Counter&Latch/Timer1 ==
  incrcondition : Inport
  incrvalue : Inport  Port=2
  decrcondition : Inport  Port=3
  decvalue : Inport  Port=4
  maxlimit : Inport  Port=5
  reset : Inport  Port=6
  Constant{,1..3} (4 alike) : Constant  Value=0  OutDataTypeStr=Inherit: Inherit via back propagation
  MinMax1 : MinMax  Inputs=2  OutDataTypeStr=Inherit: Inherit via back propagation  InputSameDT=on
  MinMax2 : MinMax  Function=max  Inputs=2  OutDataTypeStr=Inherit: Inherit via back propagation  InputSameDT=on
  Relational Operator : RelationalOperator  OutDataTypeStr=boolean  RndMeth=Nearest
  Sum : Sum  Inputs=++-  OutDataTypeStr=Inherit: Inherit via back propagation  InputSameDT=on
  Unit Delay : UnitDelay  SampleTime=-1
  dec switch : Switch  Criteria=u2 ~= 0  Threshold=1  OutDataTypeStr=Inherit: Inherit via back propagation  InputSameDT=on
  inc switch : Switch  Criteria=u2 ~= 0  Threshold=1  OutDataTypeStr=Inherit: Inherit via back propagation  InputSameDT=on
  reset switch : Switch  Criteria=u2 ~= 0  Threshold=1  OutDataTypeStr=Inherit: Inherit via back propagation  InputSameDT=on
  counter out : Outport
  counter_status : Outport  Port=2
  wires:
  decvalue/1 -> dec switch/1
  Relational Operator/1 -> counter_status/1
  Constant3/1 -> reset switch/1
  inc switch/1 -> Sum/2
  Sum/1 -> MinMax2/2
  maxlimit/1 -> MinMax1/2, Relational Operator/2
  Constant2/1 -> MinMax2/1
  reset switch/1 -> counter out/1, Relational Operator/1, Unit Delay/1
  Unit Delay/1 -> Sum/1
  reset/1 -> reset switch/2
  Constant/1 -> inc switch/3
  MinMax2/1 -> MinMax1/1
  incrvalue/1 -> inc switch/1
  MinMax1/1 -> reset switch/3
  dec switch/1 -> Sum/3
  Constant1/1 -> dec switch/3
  decrcondition/1 -> dec switch/2
  incrcondition/1 -> inc switch/2

== system ADIA/ADAS_Diagnostics/Diagnostics_Processing/Rationality_Diagnostics/EMS_17E_InvOorMinTrqWhl/Counter&Latch/Latch  ==
  Input : Inport
  Latch Reset : Inport  Port=2
  Constant11 : Constant  Value=0  OutDataTypeStr=Inherit: Inherit via back propagation
  Constant12 : Constant  OutDataTypeStr=Inherit: Inherit via back propagation
  Switch : Switch  Threshold=1  OutDataTypeStr=Inherit: Inherit via back propagation  SaturateOnIntegerOverflow=on  InputSameDT=on
  Switch1 : Switch  Threshold=1  OutDataTypeStr=Inherit: Inherit via back propagation  SaturateOnIntegerOverflow=on  InputSameDT=on
  Unit Delay1 : UnitDelay  SampleTime=-1
  Output : Outport  InitialOutput=0
  wires:
  Constant12/1 -> Switch1/1
  Constant11/1 -> Switch/1
  Input/1 -> Switch1/2
  Unit Delay1/1 -> Switch1/3
  Switch/1 -> Unit Delay1/1, Output/1
  Latch Reset/1 -> Switch/2
  Switch1/1 -> Switch/3

== system ADIA/ADAS_Diagnostics/Diagnostics_Processing/Rationality_Diagnostics/EMS_17E_InvOorMinTrqWhl/Counter&Latch/Timer1 ==
  incrcondition : Inport
  incrvalue : Inport  Port=2
  decrcondition : Inport  Port=3
  decvalue : Inport  Port=4
  maxlimit : Inport  Port=5
  reset : Inport  Port=6
  Constant{,1..3} (4 alike) : Constant  Value=0  OutDataTypeStr=Inherit: Inherit via back propagation
  MinMax1 : MinMax  Inputs=2  OutDataTypeStr=Inherit: Inherit via back propagation  InputSameDT=on
  MinMax2 : MinMax  Function=max  Inputs=2  OutDataTypeStr=Inherit: Inherit via back propagation  InputSameDT=on
  Relational Operator : RelationalOperator  OutDataTypeStr=boolean  RndMeth=Nearest
  Sum : Sum  Inputs=++-  OutDataTypeStr=Inherit: Inherit via back propagation  InputSameDT=on
  Unit Delay : UnitDelay  SampleTime=-1
  dec switch : Switch  Criteria=u2 ~= 0  Threshold=1  OutDataTypeStr=Inherit: Inherit via back propagation  InputSameDT=on
  inc switch : Switch  Criteria=u2 ~= 0  Threshold=1  OutDataTypeStr=Inherit: Inherit via back propagation  InputSameDT=on
  reset switch : Switch  Criteria=u2 ~= 0  Threshold=1  OutDataTypeStr=Inherit: Inherit via back propagation  InputSameDT=on
  counter out : Outport
  counter_status : Outport  Port=2
  wires:
  decvalue/1 -> dec switch/1
  Relational Operator/1 -> counter_status/1
  Constant3/1 -> reset switch/1
  inc switch/1 -> Sum/2
  Sum/1 -> MinMax2/2
  maxlimit/1 -> MinMax1/2, Relational Operator/2
  Constant2/1 -> MinMax2/1
  reset switch/1 -> counter out/1, Relational Operator/1, Unit Delay/1
  Unit Delay/1 -> Sum/1
  reset/1 -> reset switch/2
  Constant/1 -> inc switch/3
  MinMax2/1 -> MinMax1/1
  incrvalue/1 -> inc switch/1
  MinMax1/1 -> reset switch/3
  dec switch/1 -> Sum/3
  Constant1/1 -> dec switch/3
  decrcondition/1 -> dec switch/2
  incrcondition/1 -> inc switch/2

== system ADIA/ADAS_Diagnostics/Diagnostics_Processing/Rationality_Diagnostics/EPS2_17A_InvOorSteAngle/Counter&Latch/Latch  ==
  Input : Inport
  Latch Reset : Inport  Port=2
  Constant11 : Constant  Value=0  OutDataTypeStr=Inherit: Inherit via back propagation
  Constant12 : Constant  OutDataTypeStr=Inherit: Inherit via back propagation
  Switch : Switch  Threshold=1  OutDataTypeStr=Inherit: Inherit via back propagation  SaturateOnIntegerOverflow=on  InputSameDT=on
  Switch1 : Switch  Threshold=1  OutDataTypeStr=Inherit: Inherit via back propagation  SaturateOnIntegerOverflow=on  InputSameDT=on
  Unit Delay1 : UnitDelay  SampleTime=-1
  Output : Outport  InitialOutput=0
  wires:
  Constant12/1 -> Switch1/1
  Constant11/1 -> Switch/1
  Input/1 -> Switch1/2
  Unit Delay1/1 -> Switch1/3
  Switch/1 -> Unit Delay1/1, Output/1
  Latch Reset/1 -> Switch/2
  Switch1/1 -> Switch/3

== system ADIA/ADAS_Diagnostics/Diagnostics_Processing/Rationality_Diagnostics/EPS2_17A_InvOorSteAngle/Counter&Latch/Timer1 ==
  incrcondition : Inport
  incrvalue : Inport  Port=2
  decrcondition : Inport  Port=3
  decvalue : Inport  Port=4
  maxlimit : Inport  Port=5
  reset : Inport  Port=6
  Constant{,1..3} (4 alike) : Constant  Value=0  OutDataTypeStr=Inherit: Inherit via back propagation
  MinMax1 : MinMax  Inputs=2  OutDataTypeStr=Inherit: Inherit via back propagation  InputSameDT=on
  MinMax2 : MinMax  Function=max  Inputs=2  OutDataTypeStr=Inherit: Inherit via back propagation  InputSameDT=on
  Relational Operator : RelationalOperator  OutDataTypeStr=boolean  RndMeth=Nearest
  Sum : Sum  Inputs=++-  OutDataTypeStr=Inherit: Inherit via back propagation  InputSameDT=on
  Unit Delay : UnitDelay  SampleTime=-1
  dec switch : Switch  Criteria=u2 ~= 0  Threshold=1  OutDataTypeStr=Inherit: Inherit via back propagation  InputSameDT=on
  inc switch : Switch  Criteria=u2 ~= 0  Threshold=1  OutDataTypeStr=Inherit: Inherit via back propagation  InputSameDT=on
  reset switch : Switch  Criteria=u2 ~= 0  Threshold=1  OutDataTypeStr=Inherit: Inherit via back propagation  InputSameDT=on
  counter out : Outport
  counter_status : Outport  Port=2
  wires:
  decvalue/1 -> dec switch/1
  Relational Operator/1 -> counter_status/1
  Constant3/1 -> reset switch/1
  inc switch/1 -> Sum/2
  Sum/1 -> MinMax2/2
  maxlimit/1 -> MinMax1/2, Relational Operator/2
  Constant2/1 -> MinMax2/1
  reset switch/1 -> counter out/1, Relational Operator/1, Unit Delay/1
  Unit Delay/1 -> Sum/1
  reset/1 -> reset switch/2
  Constant/1 -> inc switch/3
  MinMax2/1 -> MinMax1/1
  incrvalue/1 -> inc switch/1
  MinMax1/1 -> reset switch/3
  dec switch/1 -> Sum/3
  Constant1/1 -> dec switch/3
  decrcondition/1 -> dec switch/2
  incrcondition/1 -> inc switch/2

== system ADIA/ADAS_Diagnostics/Diagnostics_Processing/Rationality_Diagnostics/EPS2_17A_InvStTorq/Counter&Latch/Latch  ==
  Input : Inport
  Latch Reset : Inport  Port=2
  Constant11 : Constant  Value=0  OutDataTypeStr=Inherit: Inherit via back propagation
  Constant12 : Constant  OutDataTypeStr=Inherit: Inherit via back propagation
  Switch : Switch  Threshold=1  OutDataTypeStr=Inherit: Inherit via back propagation  SaturateOnIntegerOverflow=on  InputSameDT=on
  Switch1 : Switch  Threshold=1  OutDataTypeStr=Inherit: Inherit via back propagation  SaturateOnIntegerOverflow=on  InputSameDT=on
  Unit Delay1 : UnitDelay  SampleTime=-1
  Output : Outport  InitialOutput=0
  wires:
  Constant12/1 -> Switch1/1
  Constant11/1 -> Switch/1
  Input/1 -> Switch1/2
  Unit Delay1/1 -> Switch1/3
  Switch/1 -> Unit Delay1/1, Output/1
  Latch Reset/1 -> Switch/2
  Switch1/1 -> Switch/3

== system ADIA/ADAS_Diagnostics/Diagnostics_Processing/Rationality_Diagnostics/EPS2_17A_InvStTorq/Counter&Latch/Timer1 ==
  incrcondition : Inport
  incrvalue : Inport  Port=2
  decrcondition : Inport  Port=3
  decvalue : Inport  Port=4
  maxlimit : Inport  Port=5
  reset : Inport  Port=6
  Constant{,1..3} (4 alike) : Constant  Value=0  OutDataTypeStr=Inherit: Inherit via back propagation
  MinMax1 : MinMax  Inputs=2  OutDataTypeStr=Inherit: Inherit via back propagation  InputSameDT=on
  MinMax2 : MinMax  Function=max  Inputs=2  OutDataTypeStr=Inherit: Inherit via back propagation  InputSameDT=on
  Relational Operator : RelationalOperator  OutDataTypeStr=boolean  RndMeth=Nearest
  Sum : Sum  Inputs=++-  OutDataTypeStr=Inherit: Inherit via back propagation  InputSameDT=on
  Unit Delay : UnitDelay  SampleTime=-1
  dec switch : Switch  Criteria=u2 ~= 0  Threshold=1  OutDataTypeStr=Inherit: Inherit via back propagation  InputSameDT=on
  inc switch : Switch  Criteria=u2 ~= 0  Threshold=1  OutDataTypeStr=Inherit: Inherit via back propagation  InputSameDT=on
  reset switch : Switch  Criteria=u2 ~= 0  Threshold=1  OutDataTypeStr=Inherit: Inherit via back propagation  InputSameDT=on
  counter out : Outport
  counter_status : Outport  Port=2
  wires:
  decvalue/1 -> dec switch/1
  Relational Operator/1 -> counter_status/1
  Constant3/1 -> reset switch/1
  inc switch/1 -> Sum/2
  Sum/1 -> MinMax2/2
  maxlimit/1 -> MinMax1/2, Relational Operator/2
  Constant2/1 -> MinMax2/1
  reset switch/1 -> counter out/1, Relational Operator/1, Unit Delay/1
  Unit Delay/1 -> Sum/1
  reset/1 -> reset switch/2
  Constant/1 -> inc switch/3
  MinMax2/1 -> MinMax1/1
  incrvalue/1 -> inc switch/1
  MinMax1/1 -> reset switch/3
  dec switch/1 -> Sum/3
  Constant1/1 -> dec switch/3
  decrcondition/1 -> dec switch/2
  incrcondition/1 -> inc switch/2

== system ADIA/ADAS_Diagnostics/Diagnostics_Processing/Rationality_Diagnostics/EPS3_31C_InvOorLKAState/Counter&Latch/Latch  ==
  Input : Inport
  Latch Reset : Inport  Port=2
  Constant11 : Constant  Value=0  OutDataTypeStr=Inherit: Inherit via back propagation
  Constant12 : Constant  OutDataTypeStr=Inherit: Inherit via back propagation
  Switch : Switch  Threshold=1  OutDataTypeStr=Inherit: Inherit via back propagation  SaturateOnIntegerOverflow=on  InputSameDT=on
  Switch1 : Switch  Threshold=1  OutDataTypeStr=Inherit: Inherit via back propagation  SaturateOnIntegerOverflow=on  InputSameDT=on
  Unit Delay1 : UnitDelay  SampleTime=-1
  Output : Outport  InitialOutput=0
  wires:
  Constant12/1 -> Switch1/1
  Constant11/1 -> Switch/1
  Input/1 -> Switch1/2
  Unit Delay1/1 -> Switch1/3
  Switch/1 -> Unit Delay1/1, Output/1
  Latch Reset/1 -> Switch/2
  Switch1/1 -> Switch/3

== system ADIA/ADAS_Diagnostics/Diagnostics_Processing/Rationality_Diagnostics/EPS3_31C_InvOorLKAState/Counter&Latch/Timer1 ==
  incrcondition : Inport
  incrvalue : Inport  Port=2
  decrcondition : Inport  Port=3
  decvalue : Inport  Port=4
  maxlimit : Inport  Port=5
  reset : Inport  Port=6
  Constant{,1..3} (4 alike) : Constant  Value=0  OutDataTypeStr=Inherit: Inherit via back propagation
  MinMax1 : MinMax  Inputs=2  OutDataTypeStr=Inherit: Inherit via back propagation  InputSameDT=on
  MinMax2 : MinMax  Function=max  Inputs=2  OutDataTypeStr=Inherit: Inherit via back propagation  InputSameDT=on
  Relational Operator : RelationalOperator  OutDataTypeStr=boolean  RndMeth=Nearest
  Sum : Sum  Inputs=++-  OutDataTypeStr=Inherit: Inherit via back propagation  InputSameDT=on
  Unit Delay : UnitDelay  SampleTime=-1
  dec switch : Switch  Criteria=u2 ~= 0  Threshold=1  OutDataTypeStr=Inherit: Inherit via back propagation  InputSameDT=on
  inc switch : Switch  Criteria=u2 ~= 0  Threshold=1  OutDataTypeStr=Inherit: Inherit via back propagation  InputSameDT=on
  reset switch : Switch  Criteria=u2 ~= 0  Threshold=1  OutDataTypeStr=Inherit: Inherit via back propagation  InputSameDT=on
  counter out : Outport
  counter_status : Outport  Port=2
  wires:
  decvalue/1 -> dec switch/1
  Relational Operator/1 -> counter_status/1
  Constant3/1 -> reset switch/1
  inc switch/1 -> Sum/2
  Sum/1 -> MinMax2/2
  maxlimit/1 -> MinMax1/2, Relational Operator/2
  Constant2/1 -> MinMax2/1
  reset switch/1 -> counter out/1, Relational Operator/1, Unit Delay/1
  Unit Delay/1 -> Sum/1
  reset/1 -> reset switch/2
  Constant/1 -> inc switch/3
  MinMax2/1 -> MinMax1/1
  incrvalue/1 -> inc switch/1
  MinMax1/1 -> reset switch/3
  dec switch/1 -> Sum/3
  Constant1/1 -> dec switch/3
  decrcondition/1 -> dec switch/2
  incrcondition/1 -> inc switch/2
